simulink model "q_srv02_mdl"  (Simulink 7.0)
settings: Solver=ode1  StartTime=0.0  StopTime=5  FixedStep=0.001  RelTol=1e-3  AbsTol=1e-6
values from neighbouring files (symbols this model uses):
  K = Am / Beq_v    [d_model_param.m]    (also in setup_srv02_exp01_mdl.m = 1)
  K_CABLE = 1    [setup_srv02_exp01_mdl.m]
  K_ENC = 0    [config_srv02.m]
  K_POT = -(352 * pi / 180 / 10)    (= -0.614355896702)    [config_srv02.m]
  K_TACH = -(1000 * 2 * pi / 60 / 1.5 / Kg)    [config_srv02.m]
  tau = Jeq / Beq_v    [d_model_param.m]    (also in setup_srv02_exp01_mdl.m = 0.1)
  VMAX_DAC = 10    [setup_srv02_exp01_mdl.m]
  VMAX_UPM = 0    [config_srv02.m]
  wcf_e = 2 * pi * 25.0    (= 157.079632679)    [setup_srv02_exp01_mdl.m]
  zetaf_e = 0.9    [setup_srv02_exp01_mdl.m]
undefined symbols (not defined in the file or in its folder): HIL, qc_get_step_size
libraries: quarc_library x5, simulink x2, simulink_extras x1
settings Model: Creator=MLevis  LastModifiedBy=FKhan  SimulationMode=external  ExtModeTrigDuration=10000  BufferReuse=off
settings SolverCC: PositivePriorityOrder=on
settings DataIOCC: LimitDataPoints=off
settings OptimizationCC: BlockReduction=off  BooleanDataType=off  InlineInvariantSignals=on  OptimizeBlockIOStorage=off  BufferReuse=off  ExpressionFolding=off  LocalBlockOutputs=off
settings DebuggingCC: SaveWithParameterizedLinksMsg=none  SignalResolutionControl=TryResolveAllWithWarning  SolverPrmCheckMsg=none  MultiTaskDSMMsg=warning  MultiTaskCondExecSysMsg=none  StrictBusMsg=None
settings HardwareCC: TargetHWDeviceType=32-bit Generic
settings RTWCC: SystemTargetFile=quarc_windows.tlc  TemplateMakefile=quarc_default_tmf  Description=Quarc Win32 Target  ProcessScript=quarc_windows_make_rtw_hook  IncludeERTFirstTime=on
settings STFCustomTargetCC: TargetFcnLib=ansi_tfl_tmw.mat  TargetPreCompLibLocation=C:\DOCUME~1\ALLUSE~1\APPLIC~1\QuaRC\lib\2007b\windows\release  GenFloatMathFcnCalls=ANSI_C  SystemTargetFile=quarc_windows.tlc
settings GRTTargetCC: TargetFcnLib=ansi_tfl_tmw.mat  TargetPreCompLibLocation=C:\DOCUME~1\ALLUSE~1\APPLIC~1\QuaRC\lib\2007b\windows\release  CompOptLevelCompliant=off  MatFileLogging=off  ExtMode=on  ExtModeMexFile=quarc_comm

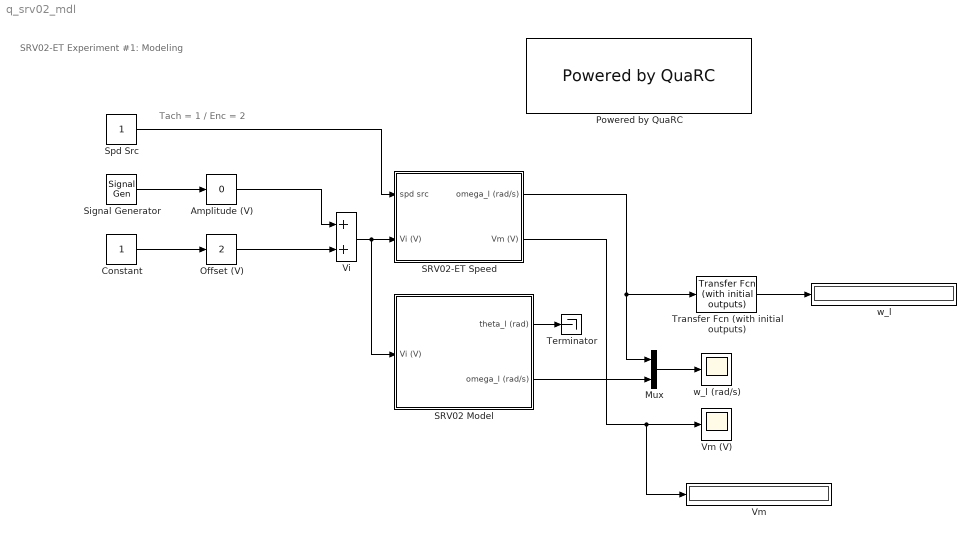
== system q_srv02_mdl ==
  note: SRV02-ET Experiment #1: Modeling
  note: Tach = 1 / Enc = 2
  Amplitude (V) : simulink/Math Operations/Slider Gain  SystemSampleTime=-1  low=0  gain=0  high=5
  Constant : Constant  OutDataType=sfix(16)  OutScaling=2^0
  Mux : Mux  Inputs=2
  Offset (V) : simulink/Math Operations/Slider Gain  SystemSampleTime=-1  low=-5  gain=2  high=5
  Powered by QuaRC : quarc_library/Logos/Powered by QuaRC  SystemSampleTime=-1
  SRV02 Model : Subsystem
  SRV02-ET Speed : Subsystem
  Signal Generator : SignalGenerator  Amplitude=0
  Spd Src : Constant  OutDataType=sfix(16)  OutScaling=2^0
  Terminator : Terminator
  Transfer Fcn (with initial outputs) : simulink_extras/Additional Linear/Transfer Fcn (with initial outputs)  SystemSampleTime=-1  N=[1]  D="[1  1]"  Y0=.5  U0=0
  Vi : Sum  OutDataType=sfix(16)  OutScaling=2^-10
  Vm : Display
      settings: Decimation=100
  Vm (V) : Scope
      settings: TimeRange=5  SaveName=Vm  DataFormat=Array
  w_l : Display
      settings: Decimation=100
  w_l (rad/s) : Scope
      settings: TimeRange=5  YMin=-3.5  YMax=3.5  SaveName=wl  DataFormat=Array
  wires:
  Constant/1 -> Offset (V)/1
  Offset (V)/1 -> Vi/2
  Vi/1 -> SRV02 Model/1(Vi (V)), SRV02-ET Speed/2(Vi (V))
  Mux/1 -> w_l (rad/s)/1
  SRV02-ET Speed/2(Vm (V)) -> Vm (V)/1, Vm/1
  SRV02 Model/2(omega_l (rad/s)) -> Mux/2
  SRV02-ET Speed/1(omega_l (rad/s)) -> Mux/1, Transfer Fcn (with initial outputs)/1
  SRV02 Model/1(theta_l (rad)) -> Terminator/1
  Signal Generator/1 -> Amplitude (V)/1
  Amplitude (V)/1 -> Vi/1
  Spd Src/1 -> SRV02-ET Speed/1(spd src)
  Transfer Fcn (with initial outputs)/1 -> w_l/1

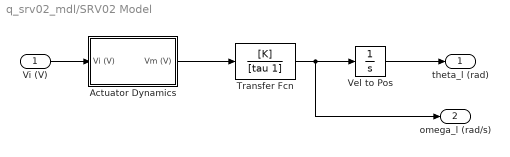
== system q_srv02_mdl/SRV02 Model ==
  Vi (V) : Inport  OutDataType=sfix(16)  OutScaling=2^0
  Actuator Dynamics : Subsystem
  Transfer Fcn : TransferFcn  Numerator=[K]  Denominator=[tau 1]
  Vel to Pos : Integrator
  theta_l (rad) : Outport  OutDataType=sfix(16)  OutScaling=2^0
  omega_l (rad/s) : Outport  Port=2  OutDataType=sfix(16)  OutScaling=2^0
  wires:
  Vi (V)/1 -> Actuator Dynamics/1(Vi (V))
  Actuator Dynamics/1(Vm (V)) -> Transfer Fcn/1
  Vel to Pos/1 -> theta_l (rad)/1
  Transfer Fcn/1 -> Vel to Pos/1, omega_l (rad/s)/1

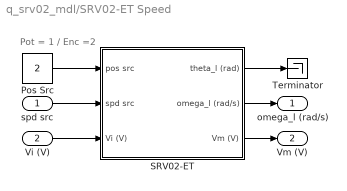
== system q_srv02_mdl/SRV02-ET Speed ==
  note: Pot = 1 / Enc =2
  spd src : Inport  OutDataType=sfix(16)  OutScaling=2^0
  Vi (V) : Inport  Port=2  OutDataType=sfix(16)  OutScaling=2^0
  Pos Src : Constant  Value=2  OutDataType=sfix(16)  OutScaling=2^0
  SRV02-ET : Subsystem
  Terminator : Terminator
  omega_l (rad/s) : Outport  OutDataType=sfix(16)  OutScaling=2^0
  Vm (V) : Outport  Port=2  OutDataType=sfix(16)  OutScaling=2^0
  wires:
  SRV02-ET/3(Vm (V)) -> Vm (V)/1
  Vi (V)/1 -> SRV02-ET/3(Vi (V))
  SRV02-ET/2(omega_l (rad/s)) -> omega_l (rad/s)/1
  spd src/1 -> SRV02-ET/2(spd src)
  SRV02-ET/1(theta_l (rad)) -> Terminator/1
  Pos Src/1 -> SRV02-ET/1(pos src)

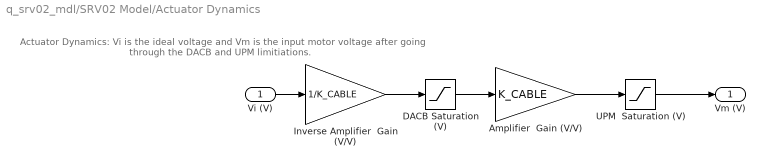
== system q_srv02_mdl/SRV02 Model/Actuator Dynamics ==
  note: Actuator Dynamics: Vi is the ideal voltage and Vm is the
      | input motor voltage after going through the DACB and UPM limitiations.
  Vi (V) : Inport  OutDataType=sfix(16)  OutScaling=2^0
  Amplifier  Gain (V/V) : Gain  Gain=K_CABLE  ParameterDataType=sfix(16)  ParameterScaling=2^0  OutDataType=sfix(16)  OutScaling=2^0
  DACB Saturation (V) : Saturate  UpperLimit=VMAX_DAC  LowerLimit=-VMAX_DAC
  Inverse Amplifier  Gain (V/V) : Gain  Gain=1/K_CABLE  ParameterDataType=sfix(16)  ParameterScaling=2^0  OutDataType=sfix(16)  OutScaling=2^0
  UPM  Saturation (V) : Saturate  UpperLimit=VMAX_UPM  LowerLimit=-VMAX_UPM
  Vm (V) : Outport  OutDataType=sfix(16)  OutScaling=2^0
  wires:
  Inverse Amplifier  Gain (V/V)/1 -> DACB Saturation (V)/1
  DACB Saturation (V)/1 -> Amplifier  Gain (V/V)/1
  Amplifier  Gain (V/V)/1 -> UPM  Saturation (V)/1
  Vi (V)/1 -> Inverse Amplifier  Gain (V/V)/1
  UPM  Saturation (V)/1 -> Vm (V)/1

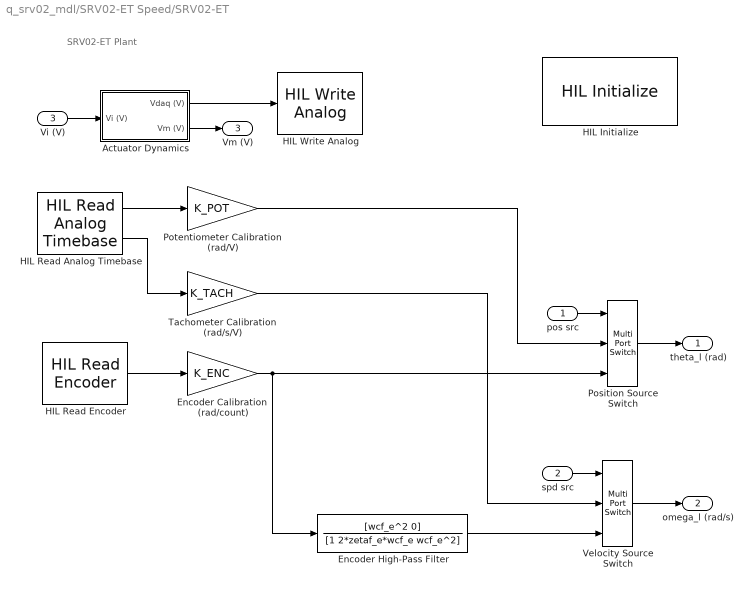
== system q_srv02_mdl/SRV02-ET Speed/SRV02-ET ==
  note: SRV02-ET Plant
  pos src : Inport  OutDataType=sfix(16)  OutScaling=2^0
  spd src : Inport  Port=2  OutDataType=sfix(16)  OutScaling=2^0
  Vi (V) : Inport  Port=3  OutDataType=sfix(16)  OutScaling=2^0
  Actuator Dynamics : Subsystem
  Encoder Calibration  (rad/count) : Gain  Gain=K_ENC  ParameterDataType=sfix(16)  ParameterScaling=2^0  OutDataType=sfix(16)  OutScaling=2^0  SaturateOnIntegerOverflow=on
  Encoder High-Pass Filter : TransferFcn  Numerator=[wcf_e^2 0]  Denominator=[1 2*zetaf_e*wcf_e wcf_e^2]
  HIL Initialize : quarc_library/Data Acquisition/Generic/Configuration/HIL Initialize  object_name=HIL-1  board_type=q8  board_number=0  active=on  hardware_clocks=0:1  clock_modes=[0 0]  set_clock_params_at_start=on  set_clock_params_at_switch_in=off  analog_input_channels=0:7  analog_input_maximums=10  analog_input_minimums=-10  set_analog_input_params_at_start=on  set_analog_input_params_at_switch_in=off  analog_output_channels=0:7  analog_output_maximums=10  analog_output_minimums=-10  initial_analog_outputs=0  final_analog_outputs=0  watchdog_analog_outputs=0  set_analog_output_params_at_start=on  set_analog_output_params_at_switch_in=off  set_analog_outputs_at_start=on  set_analog_outputs_at_switch_in=off  set_analog_outputs_at_terminate=on  set_analog_outputs_at_switch_out=off  set_analog_outputs_on_watchdog=off  digital_input_channels=[]  digital_output_channels=[]  initial_digital_outputs=1  final_digital_outputs=1  watchdog_digital_outputs=0  set_digital_outputs_at_start=on  set_digital_outputs_at_switch_in=off  set_digital_outputs_at_terminate=on  set_digital_outputs_at_switch_out=off  set_digital_outputs_on_watchdog=off  encoder_channels=0:7  quadrature=4  encoder_filter_frequency=(1/60e-9)/1  initial_encoder_counts=0  set_encoder_params_at_start=on  set_encoder_params_at_switch_in=off  set_encoder_counts_at_start=on  set_encoder_counts_at_switch_in=off  pwm_channels=[]  pwm_modes=0  pwm_frequency=(1/60e-9)/1024  initial_pwm_outputs=0  final_pwm_outputs=0  watchdog_pwm_outputs=0  set_pwm_params_at_start=on  set_pwm_params_at_switch_in=off  set_pwm_outputs_at_start=on  set_pwm_outputs_at_switch_in=off  set_pwm_outputs_at_terminate=on  set_pwm_outputs_at_switch_out=off  set_pwm_outputs_on_watchdog=off  other_output_channels=[]  initial_other_outputs=[]  final_other_outputs=[]  watchdog_other_outputs=0  set_other_outputs_at_start=on  set_other_outputs_at_switch_in=off  set_other_outputs_at_terminate=on  set_other_outputs_at_switch_out=off  set_other_outputs_on_watchdog=off
      settings: AttributesFormatString=%<object_name>
  HIL Read Analog Timebase : quarc_library/Data Acquisition/Generic/Timebases/HIL Read Analog Timebase  Tag=unassigned  object_name=HIL-1  clock=0  channels=[0,2]  samples_in_buffer=max(ceil(1/qc_get_step_size), 1)  active=on  vector_output=off
      settings: AttributesFormatString=(%<object_name>)
  HIL Read Encoder : quarc_library/Data Acquisition/Generic/Immediate I//O/HIL Read Encoder  Tag=unassigned  object_name=HIL-1  channels=0  sample_time=qc_get_step_size  active=on  vector_output=off  data_type_mode=Inherit via back propagation  data_type=double
  HIL Write Analog : quarc_library/Data Acquisition/Generic/Immediate I//O/HIL Write Analog  Tag=unassigned  object_name=HIL-1  channels=0  sample_time=-1  active=off  vector_input=off
  Position Source Switch : MultiPortSwitch  Inputs=2
  Potentiometer Calibration  (rad/V) : Gain  Gain=K_POT  ParameterDataType=sfix(16)  ParameterScaling=2^0  OutDataType=sfix(16)  OutScaling=2^0  SaturateOnIntegerOverflow=on
  Tachometer Calibration  (rad/s/V) : Gain  Gain=K_TACH  ParameterDataType=sfix(16)  ParameterScaling=2^0  OutDataType=sfix(16)  OutScaling=2^0  SaturateOnIntegerOverflow=on
  Velocity Source Switch : MultiPortSwitch  Inputs=2
  theta_l (rad) : Outport  OutDataType=sfix(16)  OutScaling=2^0  InitialOutput=0
  omega_l (rad/s) : Outport  Port=2  OutDataType=sfix(16)  OutScaling=2^0  InitialOutput=0
  Vm (V) : Outport  Port=3  OutDataType=sfix(16)  OutScaling=2^0  InitialOutput=0
  wires:
  HIL Read Analog Timebase/2 -> Tachometer Calibration  (rad/s/V)/1
  HIL Read Encoder/1 -> Encoder Calibration  (rad/count)/1
  Encoder High-Pass Filter/1 -> Velocity Source Switch/3
  Potentiometer Calibration  (rad/V)/1 -> Position Source Switch/2
  spd src/1 -> Velocity Source Switch/1
  pos src/1 -> Position Source Switch/1
  Position Source Switch/1 -> theta_l (rad)/1
  Velocity Source Switch/1 -> omega_l (rad/s)/1
  Actuator Dynamics/2(Vm (V)) -> Vm (V)/1
  Actuator Dynamics/1(Vdaq (V)) -> HIL Write Analog/1
  HIL Read Analog Timebase/1 -> Potentiometer Calibration  (rad/V)/1
  Vi (V)/1 -> Actuator Dynamics/1(Vi (V))
  Encoder Calibration  (rad/count)/1 -> Encoder High-Pass Filter/1, Position Source Switch/3
  Tachometer Calibration  (rad/s/V)/1 -> Velocity Source Switch/2

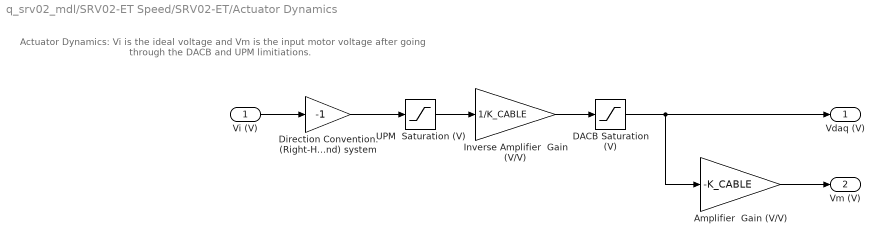
== system q_srv02_mdl/SRV02-ET Speed/SRV02-ET/Actuator Dynamics ==
  note: Actuator Dynamics: Vi is the ideal voltage and Vm is the
      | input motor voltage after going through the DACB and UPM limitiations.
  Vi (V) : Inport  OutDataType=sfix(16)  OutScaling=2^0
  Amplifier  Gain (V/V) : Gain  Gain=-K_CABLE  ParameterDataType=sfix(16)  ParameterScaling=2^0  OutDataType=sfix(16)  OutScaling=2^0
  DACB Saturation (V) : Saturate  UpperLimit=VMAX_DAC  LowerLimit=-VMAX_DAC
  Direction Convention: (Right-Hand) system : Gain  Gain=-1  ParameterDataType=sfix(16)  ParameterScaling=2^0  OutDataType=sfix(16)  OutScaling=2^0  SaturateOnIntegerOverflow=on
  Inverse Amplifier  Gain (V/V) : Gain  Gain=1/K_CABLE  ParameterDataType=sfix(16)  ParameterScaling=2^0  OutDataType=sfix(16)  OutScaling=2^0
  UPM  Saturation (V) : Saturate  UpperLimit=VMAX_UPM  LowerLimit=-VMAX_UPM
  Vdaq (V) : Outport  OutDataType=sfix(16)  OutScaling=2^0
  Vm (V) : Outport  Port=2  OutDataType=sfix(16)  OutScaling=2^0
  wires:
  Direction Convention: (Right-Hand) system/1 -> UPM  Saturation (V)/1
  Amplifier  Gain (V/V)/1 -> Vm (V)/1
  DACB Saturation (V)/1 -> Vdaq (V)/1, Amplifier  Gain (V/V)/1
  Inverse Amplifier  Gain (V/V)/1 -> DACB Saturation (V)/1
  UPM  Saturation (V)/1 -> Inverse Amplifier  Gain (V/V)/1
  Vi (V)/1 -> Direction Convention: (Right-Hand) system/1
